simulink model "BouncingBoxSimulinkProject"  (R2014b)
settings: Solver=ode45  StartTime=0.0  StopTime=20.0  RelTol=1e-3
libraries: vrlib x2
settings Model: Creator=Ben  LastModifiedBy=don

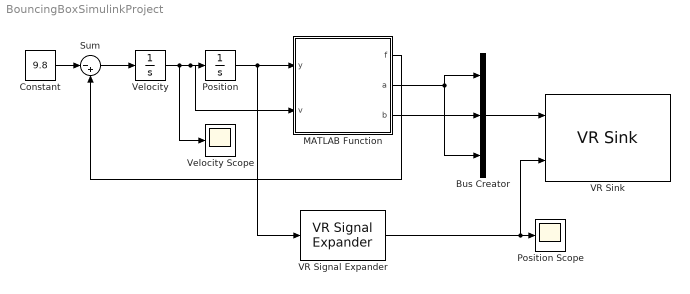
== system BouncingBoxSimulinkProject ==
  Bus Creator : BusCreator  Inputs=3
  Constant : Constant  Value=9.8
  MATLAB Function : MATLAB Function  TreatAsAtomicUnit=on
  Position : Integrator  InitialCondition=20
  Position Scope : Scope
      settings: YMin=0  YMax=20
  Sum : Sum  Inputs=|-+
  VR Signal Expander : vrlib/VR Signal Expander  outwidth=3  outidx=[2]
  VR Sink : vrlib/VR Sink  InstantiateOnLoad=on  SampleTime=0.02  ViewEnable=on  RemoteChange=off  RemoteView=on  FieldsWritten=BoxTransform.scale.3.1.1.double#BoxTransform.translation.3.1.1.double  WorldFileName=BouncingBoxSimulink.wrl  WorldDescription=VRML scene BouncingBoxSimulink.wrl  AutoView=on  VideoDimensions=[]  AllowVariableSize=off
  Velocity : Integrator
  Velocity Scope : Scope
      settings: YMin=-20  YMax=20  SaveName=ScopeData2
  wires:
  Velocity/1 -> Velocity Scope/1, MATLAB Function/2(v), Position/1
  MATLAB Function/1(f) -> Sum/2
  Constant/1 -> Sum/1
  Sum/1 -> Velocity/1
  VR Signal Expander/1 -> VR Sink/2, Position Scope/1
  MATLAB Function/2(a) -> Bus Creator/1, Bus Creator/3
  Position/1 -> VR Signal Expander/1, MATLAB Function/1(y)
  Bus Creator/1 -> VR Sink/1
  MATLAB Function/3(b) -> Bus Creator/2

== matlab function BouncingBoxSimulinkProject/MATLAB Function ==
  data: y input; f output; a output; b output; v input
% TODO add metadata

function [f, a, b] = fcn(y, v)
%#codegen
f2=0;
if y<1e-4
    y=1e-4;
end

if y<1.5  % during compression
    f1=500*(1.5-y); % spring compression equations
    if v<0 % decelerate the ball
        f2=-8*v;
    end
    a=sqrt(1.5^3/y);
    b=y;
else      % during free fall
    f1=0;
    a=1.5;
    b=1.5;
    
end 
f=f1+f2; % accumulated force
